simulink model "Esquema"  (R2018b)
settings: Solver=VariableStepAuto  StartTime=0.0  StopTime=inf  RelTol=1e-3
settings Model: Creator=alexa  LastModifiedBy=alexa

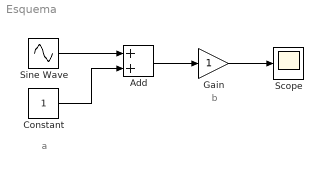
== system Esquema ==
  note: b
  note: a
  Add : Sum
  Constant : Constant
  Gain : Gain
  Scope : Scope
  Sine Wave : Sin  SampleTime=0
  wires:
  Gain/1 -> Scope/1
  Add/1 -> Gain/1
  Sine Wave/1 -> Add/1
  Constant/1 -> Add/2
